simulink model "untitled1"  (R2024a)
settings: Solver=VariableStepAuto  StartTime=0.0  StopTime=1  RelTol=1e-3
settings Model: Creator=PC  LastModifiedBy=PC

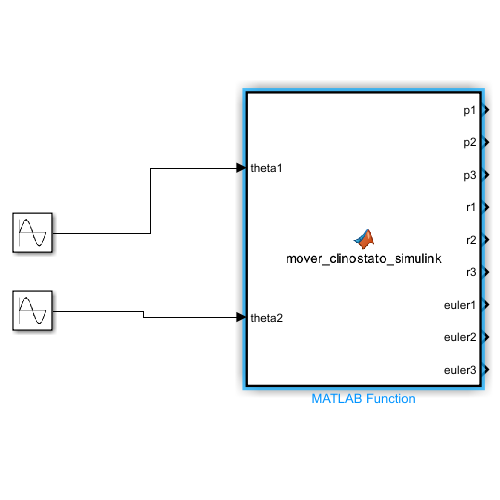
[thumbnail: Simulink's stored preview of the top-level diagram]
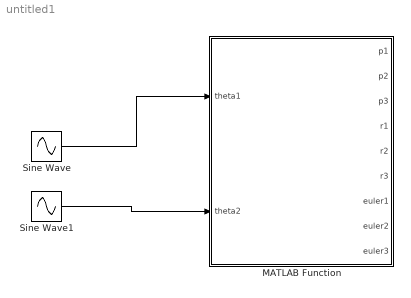
== system untitled1 ==
  MATLAB Function : MATLAB Function  TreatAsAtomicUnit=on
  Sine Wave : Sin  SampleTime=0
  Sine Wave1 : Sin  SampleTime=0
  wires:
  Sine Wave/1 -> MATLAB Function/1(theta1)
  Sine Wave1/1 -> MATLAB Function/2(theta2)

== matlab function untitled1/MATLAB Function ==
  data: theta1 input; p1 output; theta2 input; p2 output; p3 output; r1 output; r2 output; r3 output; euler1 output; euler2 output; euler3 output
function [p1, p2, p3, r1, r2, r3,euler1,euler2,euler3] = mover_clinostato_simulink( theta1, theta2)
% Llamando a la función que ya creaste
[p1, p2, p3, r1, r2, r3,euler1,euler2,euler3] = mover_clinostato_paso( theta1, theta2);
